simulink model "slew"  (R2021b)
settings: Solver=VariableStepAuto  StartTime=0.0  StopTime=T_slew  RelTol=1e-3
values from neighbouring files (symbols this model uses):
  A0 = A_end    [Project.m]
  Delta_t = T_det    (= 180)    [Project.m]
  m_max = 1e-3    (= 0.001)    [Project.m]
  momentum_storage = 1e-2    (= 0.01)    [Project.m]
  om_0 = [0.22 0.26 0.22]    [Project.m]
  pointing_accuracy = 0.5    [Project.m]
  Tm = 1/fM    (= 0.0555555555556)    [Project.m]
undefined symbols (not defined in the file or in its folder): J
settings Model: Creator=Andre  LastModifiedBy=jorgemarrero
settings SolverCC: AlgebraicLoopSolver=TrustRegion
settings DataIOCC: ReturnWorkspaceOutputs=off
settings DebuggingCC: SFMachineParentedDataDiag=warning  ArithmeticOperatorsInVariantConditions=warning
settings SFSimCC: CustomCodeUndefinedFunction=UseInterfaceOnly

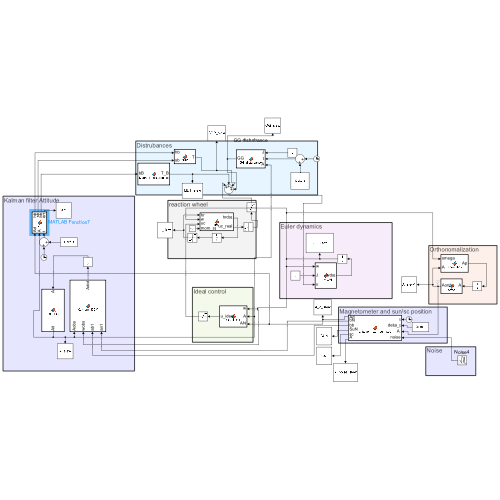
[thumbnail: Simulink's stored preview of the top-level diagram]
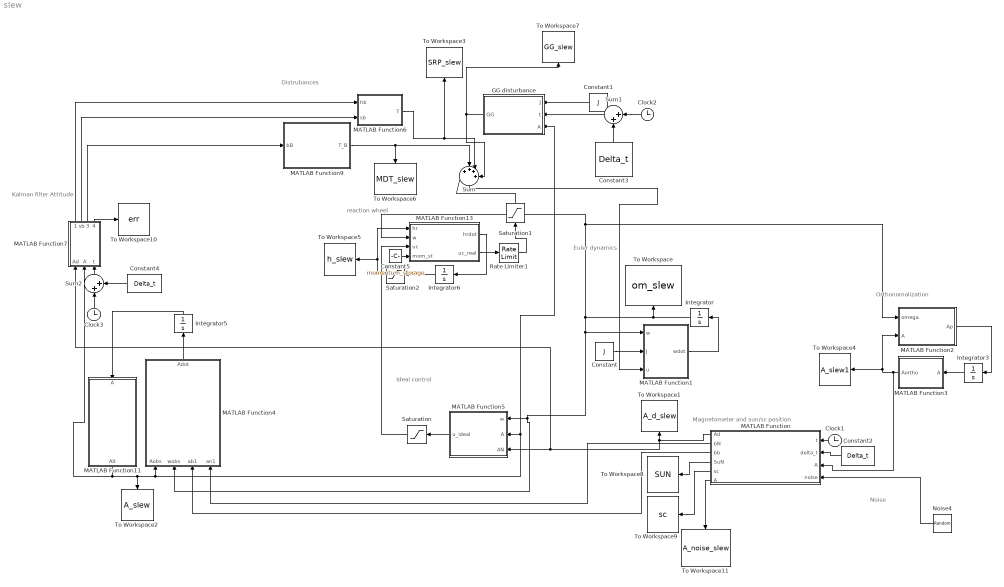
== system slew ==
  note: Magnetometer and sun/sc position
  note: Noise
  note: Distrubances
  note: Orthonomalization
  note: Euler dynamics
  note: reaction wheel
  note: Ideal control
  note: Kalman filter Attitude
  Clock1 : Clock
  Clock2 : Clock
  Clock3 : Clock
  Constant : Constant  Value=J
  Constant1 : Constant  Value=J
  Constant2 : Constant  Value=Delta_t
  Constant3 : Constant  Value=Delta_t
  Constant4 : Constant  Value=Delta_t
  Constant5 : Constant  Value=momentum_storage
  "GG disturbance " : MATLAB Function  TreatAsAtomicUnit=on
  Integrator : Integrator  InitialCondition=om_0
  Integrator3 : Integrator  InitialCondition=A0
  Integrator5 : Integrator  InitialCondition=A0
  Integrator6 : Integrator  InitialCondition=[0;0;0;0]
  MATLAB Function : MATLAB Function  TreatAsAtomicUnit=on
  MATLAB Function1 : MATLAB Function  TreatAsAtomicUnit=on
  MATLAB Function11 : MATLAB Function  TreatAsAtomicUnit=on
  MATLAB Function13 : MATLAB Function  TreatAsAtomicUnit=on
  MATLAB Function2 : MATLAB Function  TreatAsAtomicUnit=on
  MATLAB Function3 : MATLAB Function  TreatAsAtomicUnit=on
  MATLAB Function4 : MATLAB Function  TreatAsAtomicUnit=on
  MATLAB Function5 : MATLAB Function  TreatAsAtomicUnit=on
  MATLAB Function6 : MATLAB Function  TreatAsAtomicUnit=on
  MATLAB Function7 : MATLAB Function  TreatAsAtomicUnit=on
  MATLAB Function9 : MATLAB Function  TreatAsAtomicUnit=on
  Noise4 : RandomNumber  Variance=(pointing_accuracy*pi/180)^2  Seed=4  SampleTime=Tm
  Rate Limiter1 : RateLimiter  RisingSlewLimit=1e-2  FallingSlewLimit=-1e-2
  Saturation : Saturate  UpperLimit=m_max  LowerLimit=-m_max  LinearizeAsGain=off  ZeroCross=off
  Saturation1 : Saturate  UpperLimit=m_max  LowerLimit=-m_max  LinearizeAsGain=off  ZeroCross=off
  Saturation2 : Saturate  UpperLimit=momentum_storage  LowerLimit=-momentum_storage  LinearizeAsGain=off  ZeroCross=off
  Sum : Sum  Inputs=|++++
  Sum1 : Sum  Inputs=|++
  Sum2 : Sum  Inputs=|++
  To Workspace : ToWorkspace  VariableName=om_slew  SaveFormat=Timeseries  SampleTime=-1
  To Workspace1 : ToWorkspace  VariableName=A_d_slew  SaveFormat=Timeseries  SampleTime=-1
  To Workspace10 : ToWorkspace  VariableName=err  SaveFormat=Timeseries  SampleTime=-1
  To Workspace11 : ToWorkspace  VariableName=A_noise_slew  SaveFormat=Timeseries  SampleTime=-1
  To Workspace2 : ToWorkspace  VariableName=A_slew  SaveFormat=Timeseries  SampleTime=-1
  To Workspace3 : ToWorkspace  VariableName=SRP_slew  SaveFormat=Timeseries  SampleTime=-1
  To Workspace4 : ToWorkspace  VariableName=A_slew1  SaveFormat=Timeseries  SampleTime=-1
  To Workspace5 : ToWorkspace  VariableName=h_slew  SaveFormat=Timeseries  SampleTime=-1
  To Workspace6 : ToWorkspace  VariableName=MDT_slew  SaveFormat=Timeseries  SampleTime=-1
  To Workspace7 : ToWorkspace  VariableName=GG_slew  SaveFormat=Timeseries  SampleTime=-1
  To Workspace8 : ToWorkspace  VariableName=SUN  SaveFormat=Timeseries  SampleTime=-1
  To Workspace9 : ToWorkspace  VariableName=sc  SaveFormat=Timeseries  SampleTime=-1
  wires:
  Saturation2/1 -> MATLAB Function13/1(hr), To Workspace5/1
  MATLAB Function1/1(wdot) -> Integrator/1
  Constant/1 -> MATLAB Function1/2(J)
  Integrator3/1 -> MATLAB Function3/1(A)
  MATLAB Function2/1(Ap) -> Integrator3/1
  MATLAB Function3/1(Aortho) -> To Workspace4/1, MATLAB Function2/2(A), MATLAB Function/3("A ")
  Saturation/1 -> MATLAB Function13/3(uc)
  Constant1/1 -> "GG disturbance "/1(J)
  Integrator/1 -> MATLAB Function13/2(w), MATLAB Function2/1(omega), MATLAB Function1/1(w), MATLAB Function4/2(wobs), MATLAB Function5/1(w), To Workspace/1
  MATLAB Function9/1(T_B) -> To Workspace6/1, Sum/2
  MATLAB Function6/1(T) -> Sum/3, To Workspace3/1
  Sum/1 -> MATLAB Function1/3(u)
  Constant3/1 -> Sum1/2
  Clock2/1 -> Sum1/1
  Sum1/1 -> "GG disturbance "/2(t)
  Constant2/1 -> MATLAB Function/2(delta_t)
  Clock1/1 -> MATLAB Function/1(t)
  MATLAB Function11/1(Ait) -> MATLAB Function7/2(A), To Workspace2/1, MATLAB Function5/2(A), "GG disturbance "/3(A), MATLAB Function4/1(Aobs)
  Integrator5/1 -> MATLAB Function11/1(A)
  MATLAB Function4/1(Adot) -> Integrator5/1
  MATLAB Function7/3(bb) -> MATLAB Function9/1(bB)
  MATLAB Function/1(Ad) -> MATLAB Function7/1(Ad), MATLAB Function5/3(AN), To Workspace1/1
  MATLAB Function/2(bN) -> MATLAB Function4/4(an1)
  MATLAB Function/3(bb) -> MATLAB Function4/3(ab1)
  Sum2/1 -> MATLAB Function7/3(t)
  Clock3/1 -> Sum2/1
  Constant4/1 -> Sum2/2
  MATLAB Function7/2(sb) -> MATLAB Function6/2(sb)
  MATLAB Function7/1(hb) -> MATLAB Function6/1(hb)
  "GG disturbance "/1(GG) -> To Workspace7/1, Sum/4
  MATLAB Function/4(SuN) -> To Workspace8/1
  MATLAB Function/5(sc) -> To Workspace9/1
  Noise4/1 -> MATLAB Function/4(noise)
  MATLAB Function5/1(u_ideal) -> Saturation/1
  Integrator6/1 -> Saturation2/1
  Saturation1/1 -> Sum/1
  MATLAB Function7/4(err) -> To Workspace10/1
  Constant5/1 -> MATLAB Function13/4(mom_st)
  MATLAB Function13/1(hrdot) -> Integrator6/1
  MATLAB Function13/2(uc_real) -> Rate Limiter1/1
  Rate Limiter1/1 -> Saturation1/1
  MATLAB Function/6(A) -> To Workspace11/1

== matlab function slew/MATLAB Function4 ==
  data: Aobs input; wobs input; ab1 input; an1 input; Adot output
function Adot = Kalmann_DCM(Aobs,wobs,ab1,an1)
% Kalman filter for DCM:
ab1=ab1/norm(ab1);
an1=an1/norm(an1);

k1=0.1;

wmatr=[0, -wobs(3), wobs(2); wobs(3),0,-wobs(1);-wobs(2),wobs(1),0];
alfa=k1*(cross(ab1,Aobs*an1));
alfam=[0, -alfa(3), alfa(2); alfa(3),0,-alfa(1);-alfa(2),alfa(1),0];
Adot=-(wmatr+alfam)*Aobs;

== matlab function slew/MATLAB Function11 ==
  data: A input; Ait output
function Ait   = ORTHO(A)
%Orthonomalization process:
Ait= A;
for k=1:15
    
    Ait= Ait*3/2-Ait*(Ait')*Ait/2;
    
end


end

== matlab function slew/MATLAB Function13 ==
  data: hr input; w input; hrdot output; uc input; uc_real output; mom_st input
function [hrdot,uc_real] = RW(hr,w,uc,mom_st)
% Definition of the matrix A and A*:
A1 = ones(3);                % 4RW
A1 = -triu(A1,1)*1/6-tril(A1,-1)*1/6+eye(3)*5/6;
Astar = [A1;ones(1,3)*2/sqrt(3)];
A = [eye(3),ones(3,1)*1/sqrt(3)];

% Dynamics equation for the 4 reaction wheels:
hrdot = -Astar*(uc+cross(w,A*hr));
hr_mod = abs(hr);
[row,~] = find(hr_mod==mom_st) ;
if isempty(row) == 0
hhrdot = -Astar*cross(w,A*hr);
hrdot(row) = hhrdot(row);
end

uc_real = -cross(w,A*hr) - A*hrdot;

== matlab function slew/MATLAB Function1 ==
  data: w input; wdot output; J input; u input
function wdot = Euler_eq(w,J,u)

% Euler equations:

Ix=J(1);
Iy=J(2);
Iz=J(3);

A = (Iy-Iz)/Ix; 
B = (Iz-Ix)/Iy;
C= (Ix-Iy)/Iz;


wdot = [A*w(2)*w(3)+u(1)/Ix;
    B*w(1)*w(3)+u(2)/Iy; 
    C*w(2)*w(1)+u(3)/Iz];

== matlab function slew/MATLAB Function ==
  data: t input; delta_t input; Ad output; bN output; bb output; A input; noise input; SuN output; sc output; A output
function [Ad,bN,bb,SuN,sc,A] = attitude_magn_sun_pos(t,delta_t,A,noise)
%Delay+time of integration:
t=t+delta_t;
% definition of constans of the Earth and Sun
n=2*pi/(365.25*3600*24); 
B=pi/6;
ep=23.45*pi/180; % Ecliptic inclination
mu=398600;
R_sc=42164;
R_sun=149600000;
R=6371;
ne=sqrt(mu/R_sc^3);
% definition of A_desired
 SuN=R_sun*[cos(n*delta_t+B); sin(n*delta_t+B)*cos(ep); sin(n*delta_t+B)*sin(ep)];
 sc=-R_sc*[cos(ne*delta_t);sin(ne*delta_t);0];
 x1=SuN+sc;
 x1=x1/norm(x1);
 VSN=R_sun*n*[-sin(n*delta_t+B); cos(n*delta_t+B)*cos(ep); cos(n*delta_t+B)*sin(ep)];
 Vs=-R_sc*ne*[-sin(ne*delta_t);cos(ne*delta_t);0];
 Vsc=VSN+Vs;
%  Vsc=Vsc/norm(Vsc);
 x3=cross(SuN+sc,Vsc);
 x3=x3/norm(x3);
 x2=cross(x3,x1);
 x2=x2/norm(x2);
 Ad=[x1';x2';x3'];
% bb noisy:
 m=[sin(11.5*pi/180)*cos(ne*t);sin(11.5*pi/180)*sin(ne*t);cos(11.5*pi/180)];
g10=-29615*10^-9;
g11=-1728*10^-9;
h11=5186*10^-9;
H0=sqrt(g10^2+g11^2+h11^2);
rmod=42164;
rnorm=[cos(ne*t);sin(ne*t);0];
bN=(R^3*H0/(rmod^3))*(3*(dot(m,rnorm)*rnorm)-m);
% matrix error+noise contribution:
epsy=noise;
Aeps=[cos(epsy)*cos(epsy), cos(epsy)*sin(epsy)*sin(epsy)+sin(epsy)*cos(epsy),-cos(epsy)*sin(epsy)*cos(epsy)+sin(epsy)*sin(epsy); 
    -sin(epsy)*cos(epsy), -sin(epsy)*sin(epsy)*sin(epsy)+cos(epsy)*cos(epsy),sin(epsy)*sin(epsy)*cos(epsy)+cos(epsy)*sin(epsy);
   sin(epsy), -cos(epsy)*sin(epsy),cos(epsy)*cos(epsy)];
 A=A*Aeps;   
 bb=A*bN;

end

== matlab function slew/MATLAB Function2 ==
  data: omega input; Ap output; A input
function Ap = kinematics(omega,A)
%kinematic equation:
Ap=-[0, -omega(3), omega(2);omega(3), 0, -omega(1);-omega(2), omega(1), 0]*A;

end

== matlab function slew/MATLAB Function3 ==
  data: A input; Aortho output
function Aortho  = ortho(A)

for i=1:10
    A=3/2*A-A*(A')*A*1/2;
end
Aortho=A;
end

== matlab function slew/MATLAB Function7 ==
  data: Ad input; hb output; sb output; bb output; A input; t input; err output
function [hb,sb,bb,err] = fcn(Ad,A,t)
n = 2*pi/(365.25*3600*24); % Mean motion
B = pi/6;
ep = 23.45*pi/180; % Ecliptic inclination
mu = 398600;
R_sc = 42164;
R = 6371;
ne = sqrt(mu/R_sc^3);
 m = [sin(11.5*pi/180)*cos(ne*t);sin(11.5*pi/180)*sin(ne*t);cos(11.5*pi/180)];
g10 = -29615*10^-9;
g11 = -1728*10^-9;
h11 = 5186*10^-9;
H0 = sqrt(g10^2+g11^2+h11^2);
rmod = 42164;
rnorm = [cos(ne*t);sin(ne*t);0];
bN = (R^3*H0/(rmod^3))*(3*(dot(m,rnorm)*rnorm)-m);
HN = -[cos(ne*t);sin(ne*t);0];
SN = [cos(n*t+B); sin(n*t+B)*cos(ep); sin(n*t+B)*sin(ep)];
hb = A*HN;
sb = A*SN;
bb = A*bN;
err = trace(eye(3)-(A')*Ad);

== matlab function slew/GG disturbance  ==
  data: J input; GG output; t input; A input
function GG = GG_disturbance(J,t,A)
mu=398600;
R=42164;

n=sqrt(mu/R^3);
% definition of the cosines for the GG formula:
Aln=[cos(n*t), sin(n*t),0;-sin(n*t),cos(n*t),0;0,0,1];
Abl=A*(Aln');
c=Abl*[1;0;0];
%gravity gradient disturbance
GG=[3*n^2*(J(3)-J(2))*c(3)*c(2); 3*n^2*(J(1)-J(3))*c(1)*c(3);3*n^2*(J(2)-J(1))*c(2)*c(1)];

end

== matlab function slew/MATLAB Function5 ==
  data: w input; A input; AN input; u_ideal output
function u_ideal = CONTROL(w,A,AN)
K=0.005;
C=0.15;

% Error on the angular velocity
we=w;

% Error on the attitude matrix:

Ae=A*(AN');

diff=K*(Ae'-Ae);

 e=[diff(3,2); diff(1,3); diff(2,1)];

% Ideal control for the RW:
u_ideal=-e-C*we;

== matlab function slew/MATLAB Function6 ==
  data: hb input; sb input; T output
function T  = SRP(hb,sb)
% dimensions of the satellite
a=0.226;
b=0.10;
l=0.366;  
% oriented areas:
A=zeros(1,6);
A(1)=a*b;
A(4)=A(1);
A(2)=b*l;
A(5)=A(2);
A(3)=a*l;
A(6)=A(3);

n1=[1;0;0];
n2=[0;1;0];
n3=[0;0;1];
n4=-n1;
n5=-n2;
n6=-n3;
N=[n1,n2,n3,n4,n5,n6];
% Center of pressure:
cp1=a/2*n1;
cp2=b/2*n2;
cp3=l/2*n3;
cp4=-cp1;
cp5=-cp2;
cp6=-cp3;
CP=[cp1,cp2,cp3,cp4,cp5,cp6];


% Pressure calculation:
Fsun=1358;
Fearth=9.5;
c=3*10^8;

Psun=Fsun/c;
Pearth=Fearth/c;

rhos=0.5;
rhod=0.1;
Fsun=zeros(3,6);
Fearth=zeros(3,6);
F=zeros(3,6);
T=zeros(3,1);
%torque calculation:
for ii=1:6
    
    n=N(:,ii);

Fsun(:,ii)=Psun*A(ii)*dot(sb,n)*((1-rhos)*sb+(2*rhos*dot(sb,n)+2/3*rhod)*n);
Fearth(:,ii)=Pearth*A(ii)*dot(hb,n)*((1-rhos)*hb+(2*rhos*dot(hb,n)+2/3*rhod)*n);
F(:,ii)=Fsun(:,ii)+Fearth(:,ii);

if dot(n,sb)>0
    cp=CP(:,ii);
    T=T+cross(cp,F(:,ii));
end
   
end

== matlab function slew/MATLAB Function9 ==
  data: bB input; T_B output
function T_B = Magnetic_disturbance(bB)

%magnetic disturbance:
m=[0.1;0.1;0.1];
T_B=cross(m,bB);
